simulink model "invmot"  (Simulink 4.00)
settings: Solver=ode45  StartTime=0.0  StopTime=10  MaxStep=0.0001  RelTol=1e-3
settings Model: LastModifiedBy=Gui

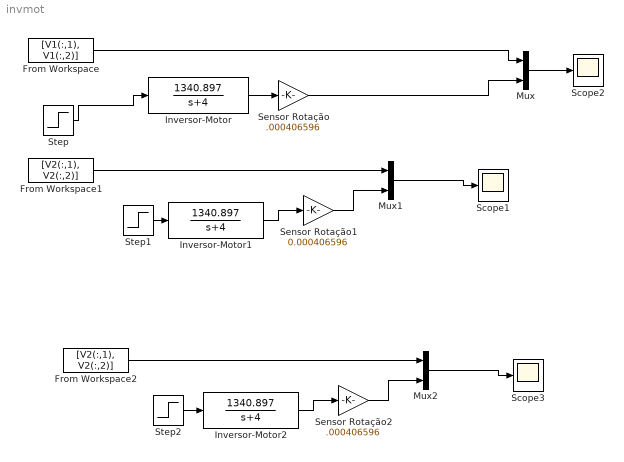
== system invmot ==
  From Workspace : FromWorkspace  VariableName=[V1(:,1), V1(:,2)]  SampleTime=0  OutputAfterFinalValue=Extrapolation
  From Workspace1 : FromWorkspace  VariableName=[V2(:,1), V2(:,2)]  SampleTime=0  OutputAfterFinalValue=Extrapolation
  From Workspace2 : FromWorkspace  VariableName=[V2(:,1), V2(:,2)]  SampleTime=0  OutputAfterFinalValue=Extrapolation
  Inversor-Motor : TransferFcn  Numerator=[1340.897]  Denominator="[1  4]"  AbsoluteTolerance=auto  Realization=auto
  Inversor-Motor1 : TransferFcn  Numerator=[1340.897]  Denominator=[1 4]  AbsoluteTolerance=auto  Realization=auto
  Inversor-Motor2 : TransferFcn  Numerator=[1340.897]  Denominator=[1 4]  AbsoluteTolerance=auto  Realization=auto
  Mux : Mux  Inputs=2
  Mux1 : Mux  Inputs=2
  Mux2 : Mux  Inputs=2
  Scope1 : Scope
      settings: TimeRange=auto  YMin=0  YMax=1  SaveToWorkspace=off  MaxDataPoints=5000
  Scope2 : Scope
      settings: TimeRange=auto  YMin=-5  YMax=5  SaveToWorkspace=off  SaveName=ScopeData  MaxDataPoints=5000
  Scope3 : Scope
      settings: TimeRange=auto  YMin=-5  YMax=5  SaveToWorkspace=off  SaveName=ScopeData2  MaxDataPoints=5000
  Sensor Rotação : Gain  Gain=.000406596  Multiplication=Element-wise(K.*u)  SaturateOnIntegerOverflow=on
  Sensor Rotação1 : Gain  Gain=0.000406596  Multiplication=Element-wise(K.*u)  SaturateOnIntegerOverflow=on
  Sensor Rotação2 : Gain  Gain=.000406596  Multiplication=Element-wise(K.*u)  SaturateOnIntegerOverflow=on
  Step : Step  Time=-8  Before=0  After=10  SampleTime=0
  Step1 : Step  Time=3.34  Before=0  After=5.223  SampleTime=0
  Step2 : Step  Time=5.65  Before=0  After=8  SampleTime=0
  wires:
  From Workspace/1 -> Mux/1
  Step/1 -> Inversor-Motor/1
  From Workspace1/1 -> Mux1/1
  Mux1/1 -> Scope1/1
  Step1/1 -> Inversor-Motor1/1
  Inversor-Motor/1 -> Sensor Rotação/1
  Inversor-Motor1/1 -> Sensor Rotação1/1
  Sensor Rotação1/1 -> Mux1/2
  Mux/1 -> Scope2/1
  Sensor Rotação/1 -> Mux/2
  From Workspace2/1 -> Mux2/1
  Mux2/1 -> Scope3/1
  Step2/1 -> Inversor-Motor2/1
  Inversor-Motor2/1 -> Sensor Rotação2/1
  Sensor Rotação2/1 -> Mux2/2
